simulink model "ElectricalDiagram"  (R2021a)
settings: Solver=VariableStepAuto  StartTime=0.0  StopTime=93*60*6+1800  RelTol=1e-3
settings Model: Creator=sarah  LastModifiedBy=sarah

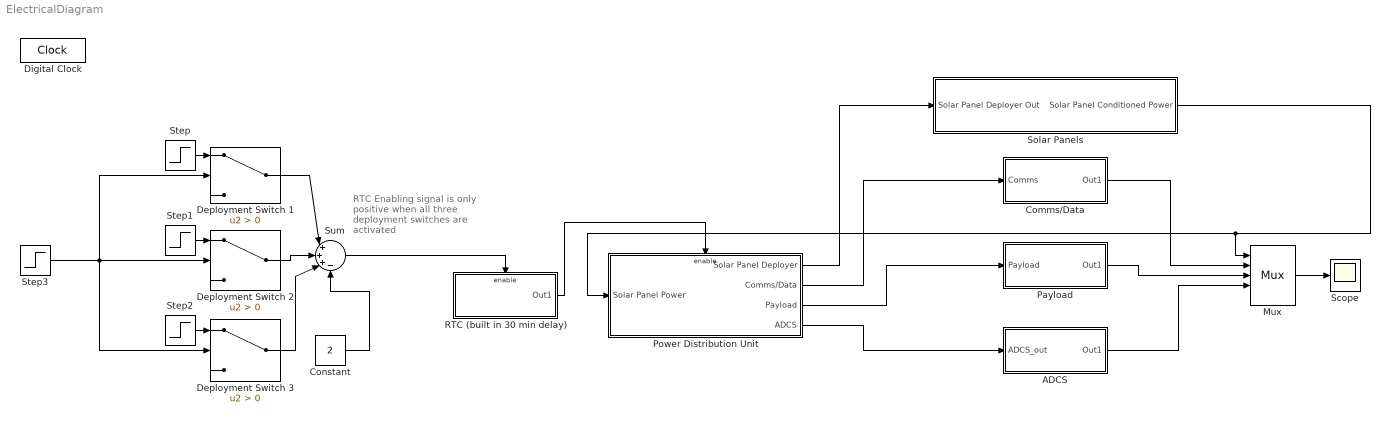
== system ElectricalDiagram ==
  note: RTC Enabling signal is only positive when all three deployment switches are activated
  ADCS : Subsystem
  Comms/Data : Subsystem
  Constant : Constant  Value=2
  Deployment Switch 1 : Switch  Criteria=u2 > Threshold
  Deployment Switch 2 : Switch  Criteria=u2 > Threshold
  Deployment Switch 3 : Switch  Criteria=u2 > Threshold
  Digital Clock : DigitalClock
  Mux : Mux  Inputs=5
  Payload : Subsystem
  Power Distribution Unit : Subsystem  TreatAsAtomicUnit=on
  RTC (built in 30 min delay) : Subsystem  TreatAsAtomicUnit=on
  Scope : Scope
  Solar Panels : Subsystem
  Step{,1..3} (4 alike) : Step  SampleTime=0
  Sum : Sum  Inputs=|+++-
  wires:
  Step/1 -> Deployment Switch 1/1
  Step1/1 -> Deployment Switch 2/1
  Step2/1 -> Deployment Switch 3/1
  Deployment Switch 1/1 -> Sum/1
  Deployment Switch 2/1 -> Sum/2
  Deployment Switch 3/1 -> Sum/3
  Step3/1 -> Deployment Switch 3/2, Deployment Switch 1/2, Deployment Switch 2/2
  Constant/1 -> Sum/4
  Sum/1 -> RTC (built in 30 min delay)/Enable
  RTC (built in 30 min delay)/1(Out1) -> Power Distribution Unit/Enable
  Solar Panels/1(Solar Panel Conditioned Power) -> Power Distribution Unit/1(Solar Panel Power), Mux/1
  Mux/1 -> Scope/1
  Comms/Data/1(Out1) -> Mux/2
  Payload/1(Out1) -> Mux/3
  ADCS/1(Out1) -> Mux/4
  Power Distribution Unit/1(Solar Panel Deployer) -> Solar Panels/1(Solar Panel Deployer Out)
  Power Distribution Unit/2(Comms/Data) -> Comms/Data/1(Comms)
  Power Distribution Unit/3(Payload) -> Payload/1(Payload)
  Power Distribution Unit/4(ADCS) -> ADCS/1(ADCS_out)

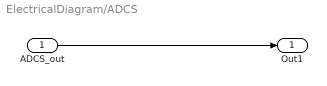
== system ElectricalDiagram/ADCS ==
  ADCS_out : Inport
  Out1 : Outport
  wires:
  ADCS_out/1 -> Out1/1

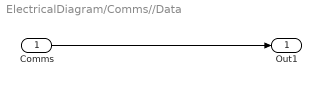
== system ElectricalDiagram/Comms//Data ==
  Comms : Inport
  Out1 : Outport
  wires:
  Comms/1 -> Out1/1

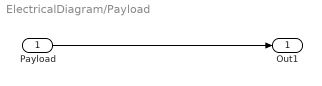
== system ElectricalDiagram/Payload ==
  Payload : Inport
  Out1 : Outport
  wires:
  Payload/1 -> Out1/1

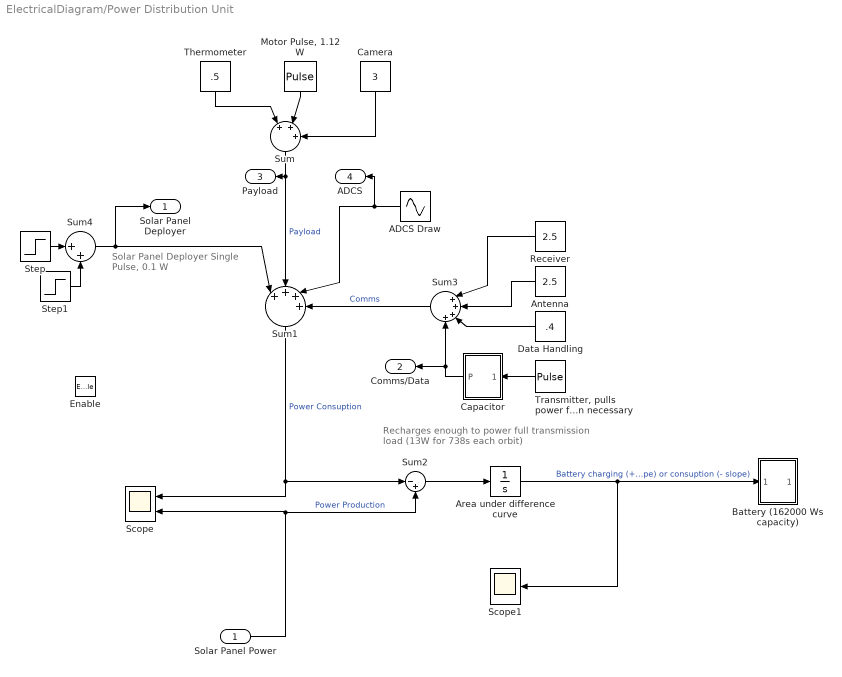
== system ElectricalDiagram/Power Distribution Unit ==
  note: Recharges enough to power full transmission load (13W for 738s each orbit)
  note: Solar Panel Deployer Single Pulse, 0.1 W
  Solar Panel Power : Inport
  Enable : EnablePort
  " Capacitor" : Subsystem
  ADCS Draw : Sin  Amplitude=.5  Bias=1  Frequency=.05  SampleTime=0
  Antenna : Constant  Value=2.5
  Area under difference curve : Integrator
  Battery (162000 Ws capacity) : Subsystem
  Camera : Constant  Value=3  VectorParams1D=off
  Data Handling : Constant  Value=.4
  "Motor Pulse, 1.12 W" : DiscretePulseGenerator  PulseType=Time based  Amplitude=.00814*3  Period=600  PulseWidth=.5
  Receiver : Constant  Value=2.5
  Scope : Scope  NumInputPorts=2
  Scope1 : Scope
  Step : Step  Time=0.025  After=.01  SampleTime=0
  Step1 : Step  Time=0.05  After=-.01  SampleTime=0
  Sum : Sum  Inputs=|+++
  Sum1 : Sum  Inputs=|++++
  Sum2 : Sum  Inputs=|-+
  Sum3 : Sum  Inputs=|++++
  Sum4 : Sum  Inputs=|++
  Thermometer : Constant  Value=.5
  "Transmitter, pulls power from capacitor when necessary" : DiscretePulseGenerator  PulseType=Time based  Amplitude=26  Period=92*60  PulseWidth=7  PhaseDelay=2600
  Solar Panel Deployer : Outport
  Comms/Data : Outport  Port=2
  Payload : Outport  Port=3
  ADCS : Outport  Port=4
  wires:
  ADCS Draw/1 -> ADCS/1, Sum1/3
  Area under difference curve/1 -> Scope1/1, Battery (162000 Ws capacity)/1(In1)  "Battery charging (+ slope) or consuption (- slope)"
  Step/1 -> Sum4/1
  " Capacitor"/1(P) -> Comms/Data/1, Sum3/4
  Camera/1 -> Sum/3
  Data Handling/1 -> Sum3/3
  Sum/1 -> Payload/1, Sum1/2  "Payload"
  Sum2/1 -> Area under difference curve/1
  Sum1/1 -> Scope/1, Sum2/1  "Power Consuption"
  Antenna/1 -> Sum3/2
  Thermometer/1 -> Sum/1
  "Transmitter, pulls power from capacitor when necessary"/1 -> " Capacitor"/1(In1)
  Step1/1 -> Sum4/2
  Sum3/1 -> Sum1/4  "Comms"
  "Motor Pulse, 1.12 W"/1 -> Sum/2
  Solar Panel Power/1 -> Scope/2, Sum2/2  "Power Production"
  Sum4/1 -> Sum1/1, Solar Panel Deployer/1
  Receiver/1 -> Sum3/1

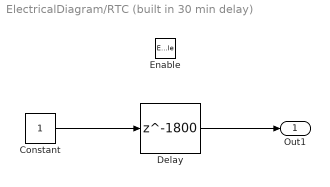
== system ElectricalDiagram/RTC (built in 30 min delay) ==
  Enable : EnablePort
  Constant : Constant
  Delay : Delay  DelayLength=1800  InitialCondition=0
  Out1 : Outport
  wires:
  Constant/1 -> Delay/1
  Delay/1 -> Out1/1

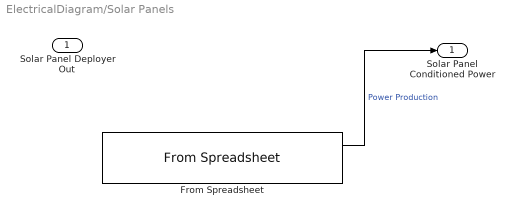
== system ElectricalDiagram/Solar Panels ==
  Solar Panel Deployer Out : Inport
  From Spreadsheet : FromSpreadsheet  FileName=SolarPanel_PowerProduction.xlsx  SheetName=SP_Power
  Solar Panel Conditioned Power : Outport
  wires:
  From Spreadsheet/1 -> Solar Panel Conditioned Power/1  "Power Production"

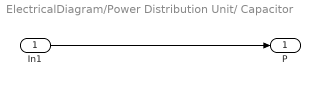
== system ElectricalDiagram/Power Distribution Unit/ Capacitor ==
  In1 : Inport
  P : Outport
  wires:
  In1/1 -> P/1

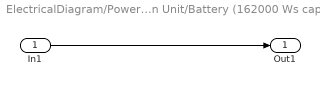
== system ElectricalDiagram/Power Distribution Unit/Battery (162000 Ws capacity) ==
  In1 : Inport
  Out1 : Outport
  wires:
  In1/1 -> Out1/1
